simulink model "modified_bouc_wen"  (R2020a)
settings: Solver=VariableStepAuto  StartTime=0.0  StopTime=10.0  RelTol=1e-3
values from neighbouring files (symbols this model uses):
  A = 301    [modified_bouc_wen_model_parameters.m]
  alpha_a = 140    [modified_bouc_wen_model_parameters.m]
  alpha_b = 695    [modified_bouc_wen_model_parameters.m]
  beta1 = 363    [modified_bouc_wen_model_parameters.m]
  c_0a = 21    [modified_bouc_wen_model_parameters.m]
  c_0b = 3.5    [modified_bouc_wen_model_parameters.m]
  c_1a = 283    [modified_bouc_wen_model_parameters.m]
  c_1b = 2.95    [modified_bouc_wen_model_parameters.m]
  eta1 = 190    [modified_bouc_wen_model_parameters.m]
  gamma1 = 363    [modified_bouc_wen_model_parameters.m]
  k0 = 46.9    [modified_bouc_wen_model_parameters.m]
  k1 = 80000    [PID_controller_tov.m]    (also in modified_bouc_wen_model_parameters.m = 5)
  n = 2    [modified_bouc_wen_model_parameters.m]
  x0 = 14.3    [modified_bouc_wen_model_parameters.m]
libraries: simulink x1
settings Model: Creator=siddh  LastModifiedBy=siddh
settings DataIOCC: ReturnWorkspaceOutputs=off

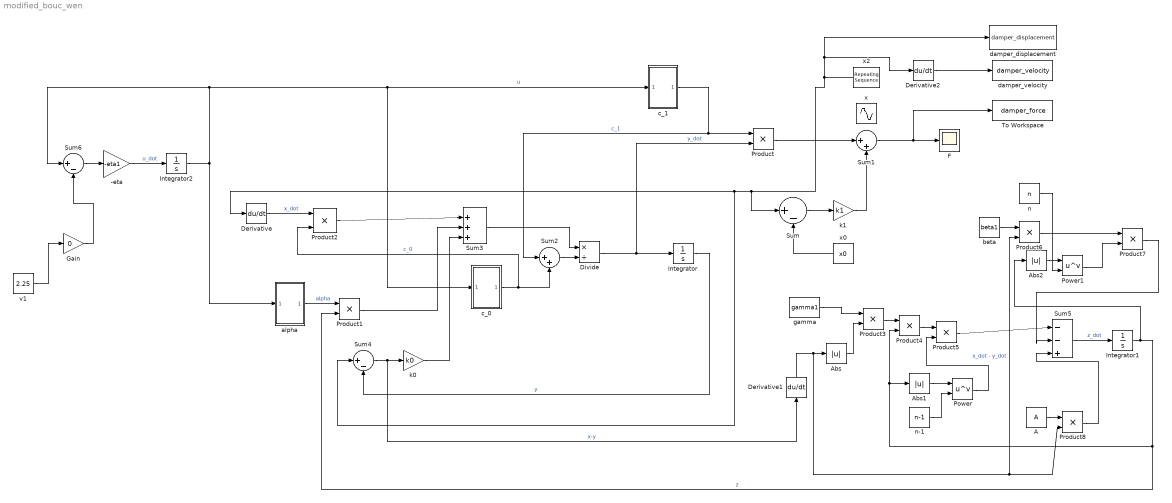
== system modified_bouc_wen ==
  -eta : Gain  Gain=-eta1
  A : Constant  Value=A
  Abs : Abs
  Abs1 : Abs
  Abs2 : Abs
  Derivative : Derivative
  Derivative1 : Derivative
  Derivative2 : Derivative
  Divide : Product  Inputs=*/
  F : Scope
  Gain : Gain  Gain=0
  Integrator : Integrator
  Integrator1 : Integrator
  Integrator2 : Integrator
  Power : Math  Operator=pow  SaturateOnIntegerOverflow=on
  Power1 : Math  Operator=pow  SaturateOnIntegerOverflow=on
  Product{,1..8} (9 alike) : Product
  Sum : Sum  Inputs=|+-
  Sum1 : Sum  Inputs=|++
  Sum2 : Sum  Inputs=|++
  Sum3 : Sum  Inputs=|+++
  Sum4 : Sum  Inputs=|+-
  Sum5 : Sum  Inputs=|--+
  Sum6 : Sum  Inputs=|+-
  To Workspace : ToWorkspace  VariableName=damper_force  SampleTime=-1
  alpha : Subsystem
  beta : Constant  Value=beta1
  c_0 : Subsystem
  c_1 : Subsystem
  damper_displacement : ToWorkspace  VariableName=damper_displacement  SampleTime=-1
  damper_velocity : ToWorkspace  VariableName=damper_velocity  SampleTime=-1
  gamma : Constant  Value=gamma1
  k0 : Gain  Gain=k0
  k1 : Gain  Gain=k1
  n : Constant  Value=n
  n-1 : Constant  Value=n-1
  v1 : Constant  Value=2.25
  x : Sin  Amplitude=0.75  Frequency=2*pi*4  SampleTime=0
  x0 : Constant  Value=x0
  x2 : simulink/Sources/Repeating Sequence  rep_seq_t=[0 0.5 1]  rep_seq_y=[0 1 0]
  wires:
  Gain/1 -> Sum6/2
  Product3/1 -> Product4/1
  x0/1 -> Sum/2
  alpha/1(Out1) -> Product1/1  "alpha"
  Sum3/1 -> Divide/1
  c_0/1(Out1) -> Product2/2, Sum2/2  "c_0"
  Abs2/1 -> Power1/1
  k0/1 -> Sum3/3
  Integrator/1 -> Sum4/2  "y"
  c_1/1(Out1) -> Product/1, Sum2/1  "c_1"
  Abs/1 -> Product3/2
  Derivative1/1 -> Product8/2, Product6/2, Abs/1  "x_dot - y_dot"
  Power/1 -> Product5/2
  Sum5/1 -> Integrator1/1  "z_dot"
  gamma/1 -> Product3/1
  -eta/1 -> Integrator2/1  "u_dot"
  Product2/1 -> Sum3/1
  Sum2/1 -> Divide/2
  Product/1 -> Sum1/1
  Derivative2/1 -> damper_velocity/1
  Sum6/1 -> -eta/1
  Integrator2/1 -> Sum6/1, c_0/1(In1), c_1/1(In1), alpha/1(In1)  "u"
  A/1 -> Product8/1
  Product4/1 -> Product5/1
  Sum/1 -> k1/1
  Product8/1 -> Sum5/3
  Integrator1/1 -> Abs2/1, Product4/2, Abs1/1, Product1/2  "z"
  v1/1 -> Gain/1
  k1/1 -> Sum1/2
  Sum1/1 -> To Workspace/1, F/1
  beta/1 -> Product6/1
  Abs1/1 -> Power/1
  Sum4/1 -> Derivative1/1, k0/1  "x-y"
  Product1/1 -> Sum3/2
  Product6/1 -> Product7/1
  n/1 -> Power1/2
  Divide/1 -> Product/2, Integrator/1  "y_dot"
  Product5/1 -> Sum5/1
  Derivative/1 -> Product2/1  "x_dot"
  Product7/1 -> Sum5/2
  Power1/1 -> Product7/2
  x2/1 -> Derivative/1, Sum4/1, Sum/1, Derivative2/1, damper_displacement/1
  n-1/1 -> Power/2

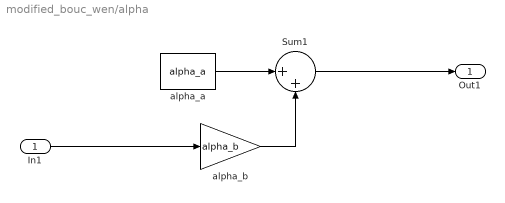
== system modified_bouc_wen/alpha ==
  In1 : Inport
  Sum1 : Sum  Inputs=|++
  alpha_a : Constant  Value=alpha_a
  alpha_b : Gain  Gain=alpha_b
  Out1 : Outport
  wires:
  In1/1 -> alpha_b/1
  alpha_b/1 -> Sum1/2
  alpha_a/1 -> Sum1/1
  Sum1/1 -> Out1/1

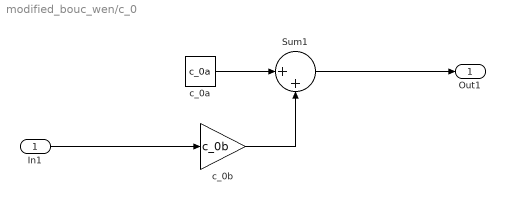
== system modified_bouc_wen/c_0 ==
  In1 : Inport
  Sum1 : Sum  Inputs=|++
  c_0a : Constant  Value=c_0a
  c_0b : Gain  Gain=c_0b
  Out1 : Outport
  wires:
  Sum1/1 -> Out1/1
  c_0a/1 -> Sum1/1
  c_0b/1 -> Sum1/2
  In1/1 -> c_0b/1

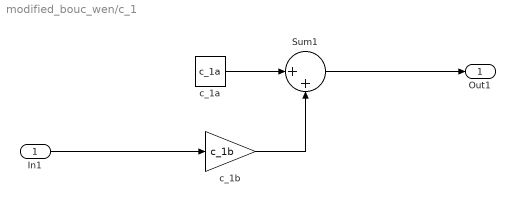
== system modified_bouc_wen/c_1 ==
  In1 : Inport
  Sum1 : Sum  Inputs=|++
  c_1a : Constant  Value=c_1a
  c_1b : Gain  Gain=c_1b
  Out1 : Outport
  wires:
  In1/1 -> c_1b/1
  c_1b/1 -> Sum1/2
  c_1a/1 -> Sum1/1
  Sum1/1 -> Out1/1
